simulink model "Simu_Design_Model_trim_LV"  (R2020a)
settings: Solver=ode45  StartTime=0.0  StopTime=10000  RelTol=1e-3  EnableMultiTasking=on
InitFcn:
  | addpath('../parameters/')
  | simulation_parameters
  | wind_parameters
  | aerosonde_parameters
  | compute_trim
undefined symbols (not defined in the file or in its folder): drawAircraft, forces_moments, plotmavstatevariables, u_trim, UAV
settings Model: Creator=beard  LastModifiedBy=h1huang
settings DataIOCC: LimitDataPoints=on  SaveFormat=Array  SignalLoggingSaveFormat=ModelDataLogs  ReturnWorkspaceOutputs=off
settings OptimizationCC: ExpressionDepthLimit=2147483647  InitFltsAndDblsToZero=on  LifeSpan=inf
settings DebuggingCC: UnderspecifiedInitializationDetection=Classic  MergeDetectMultiDrivingBlocksExec=none  SolverPrmCheckMsg=warning  FcnCallInpInsideContextMsg=warning  StateNameClashWarn=warning  SFUnexpectedBacktrackingDiag=warning  SFNoUnconditionalDefaultTransitionDiag=warning  SFExecutionAtInitializationDiag=none  ArithmeticOperatorsInVariantConditions=warning
settings HardwareCC: ProdBitPerPointer=32  ProdBitPerSizeT=32  ProdBitPerPtrDiffT=32  ProdLargestAtomicFloat=None  ProdIntDivRoundTo=Undefined  ProdEndianess=Unspecified  ProdWordSize=32  ProdHWDeviceType=32-bit Generic
settings ModelReferenceCC: PropagateSignalLabelsOutOfModel=off
settings SFSimCC: SimUseLocalCustomCode=off  CustomCodeUndefinedFunction=UseInterfaceOnly
settings RTWCC: RTWUseLocalCustomCode=off
settings CodeAppCC: StateflowObjectComments=on
settings GRTTargetCC: TargetLangStandard=C89/C90 (ANSI)  CombineOutputUpdateFcns=off  GRTInterface=on
settings ConfigComp: CovMetricSettings=dw  CovSaveCumulativeToWorkspaceVar=on  CovSaveSingleToWorkspaceVar=on  CovExternalEMLEnable=off  CovSFcnEnable=off

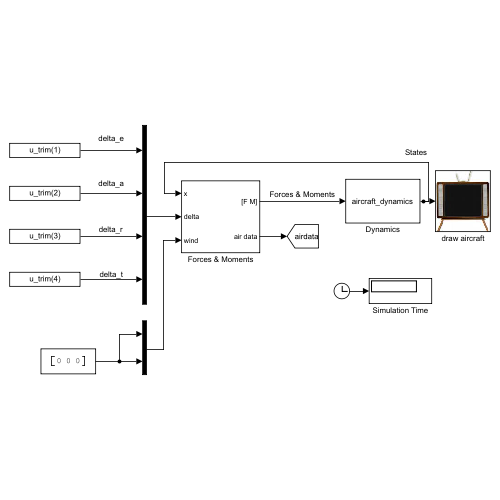
[thumbnail: Simulink's stored preview of the top-level diagram]
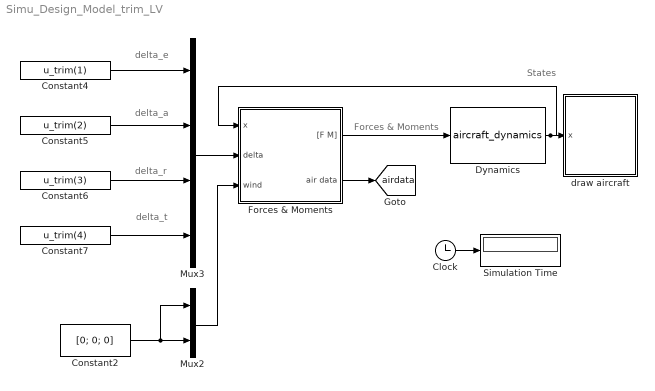
== system Simu_Design_Model_trim_LV ==
  note: delta_r
  note: delta_t
  note: Forces & Moments
  note: States
  note: delta_e
  note: delta_a
  Clock : Clock
  Constant2 : Constant  Value=[0; 0; 0]
  Constant4 : Constant  Value=u_trim(1)
  Constant5 : Constant  Value=u_trim(2)
  Constant6 : Constant  Value=u_trim(3)
  Constant7 : Constant  Value=u_trim(4)
  Dynamics : S-Function  FunctionName=aircraft_dynamics  Parameters=UAV  SFunctionDeploymentMode=off  EnableBusSupport=off
  Forces & Moments : Subsystem
  Mux2 : Mux  Inputs=2
  Mux3 : Mux
  Simulation Time : Display
  draw aircraft : Subsystem
      mask Display: image(imread('tv.jpg'))
  tag scope: airdata=global
  wires:
  Dynamics/1 -> Forces & Moments/1(x), draw aircraft/1(x)
  Forces & Moments/1("[F M]") -> Dynamics/1
  Clock/1 -> Simulation Time/1
  Forces & Moments/2(air data) -> [airdata]
  Constant2/1 -> Mux2/1, Mux2/2
  Mux3/1 -> Forces & Moments/2(delta)
  Mux2/1 -> Forces & Moments/3(wind)
  Constant4/1 -> Mux3/1
  Constant5/1 -> Mux3/2
  Constant6/1 -> Mux3/3
  Constant7/1 -> Mux3/4

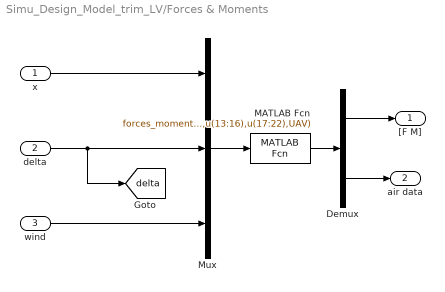
== system Simu_Design_Model_trim_LV/Forces & Moments ==
  x : Inport
  delta : Inport  Port=2
  wind : Inport  Port=3
  Demux : Demux  Outputs=[6;6]
  MATLAB Fcn : MATLABFcn  MATLABFcn=forces_moments(u(1:12),u(13:16),u(17:22),UAV)  OutputDimensions=12
  Mux : Mux  Inputs=3
  "[F M]" : Outport  VectorParamsAs1DForOutWhenUnconnected=off
  air data : Outport  Port=2  VectorParamsAs1DForOutWhenUnconnected=off
  tag scope: delta=global
  wires:
  x/1 -> Mux/1
  delta/1 -> [delta], Mux/2
  wind/1 -> Mux/3
  MATLAB Fcn/1 -> Demux/1
  Demux/1 -> "[F M]"/1
  Mux/1 -> MATLAB Fcn/1
  Demux/2 -> air data/1

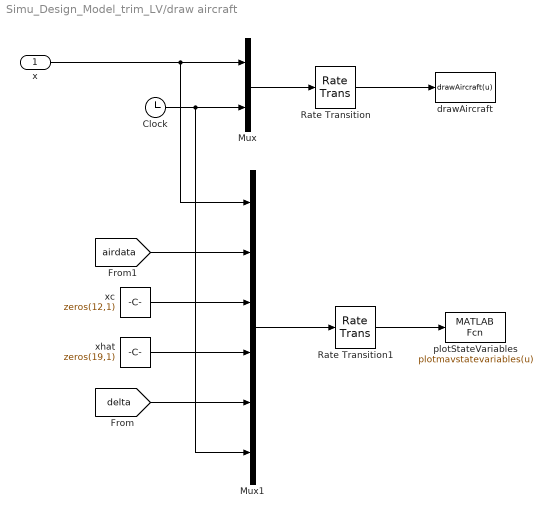
== system Simu_Design_Model_trim_LV/draw aircraft ==
  x : Inport
  Clock : Clock
  Mux : Mux  Inputs=2
  Mux1 : Mux  Inputs=6
  Rate Transition : RateTransition  OutPortSampleTime=SIM.ts_plotting
  Rate Transition1 : RateTransition  OutPortSampleTime=SIM.ts_plotting
  drawAircraft : MATLABFcn  MATLABFcn=drawAircraft(u)  OutputDimensions=0
  plotStateVariables : MATLABFcn  MATLABFcn=plotmavstatevariables(u)  OutputDimensions=0
  xc : Constant  Value=zeros(12,1)
  xhat : Constant  Value=zeros(19,1)
  wires:
  [airdata] -> Mux1/2
  [delta] -> Mux1/5
  xc/1 -> Mux1/3
  xhat/1 -> Mux1/4
  Clock/1 -> Mux1/6, Mux/2
  x/1 -> Mux1/1, Mux/1
  Rate Transition1/1 -> plotStateVariables/1
  Mux1/1 -> Rate Transition1/1
  Mux/1 -> Rate Transition/1
  Rate Transition/1 -> drawAircraft/1
